simulink model "RoboBoat_SScallv3"  (R2014a)
settings: Solver=FixedStepDiscrete  StartTime=0.0  StopTime=inf  FixedStep=.25  RelTol=1e-3
undefined symbols (not defined in the file): Com1, Com2, Com3, Com4, DiscIntNeverNeededParam, standard
libraries: xpcseriallib x31, visiontextngfix x25, simulink x19, slrtlib x9, speedgoatlib_IO102 x3, speedgoatlib x2
(part 3 of 5)

== system RoboBoat_SScallv3/Main FSM/Obstacle Navigation1/Exit Gate/Gate 1 (Red & White) ==
  Sensors : Inport
  RGB image : Inport  Port=2
  Enable : EnablePort  ShowOutputPort=on
  Bus Selector : BusSelector  OutputSignals=Serial In.Buoy Info.Probability,Serial In.Buoy Info.Color ID,Serial In.Buoy Info.Distance,Serial In.Buoy Info.Angle,Serial In.Compass.Heading,Serial In.GPS.latitude,Serial In.GPS.longitude
  Compare To Constant : simulink/Logic and Bit Operations/Compare To Constant  relop=<=  const=2  OutDataTypeStr=boolean
  Compare To Constant1 : simulink/Logic and Bit Operations/Compare To Constant  relop=>=  const=120  OutDataTypeStr=boolean
  Data Type Conversion2 : DataTypeConversion  OutDataTypeStr=double
  Discrete-Time Integrator : DiscreteIntegrator  SampleTime=.1  ICPrevOutput=DiscIntNeverNeededParam  ICPrevScaledInput=DiscIntNeverNeededParam
  Distance : MATLAB Function  TreatAsAtomicUnit=on
  Insert Text : visiontextngfix/Insert Text  inputType=Obsolete  theText='Exit Gate 1'  getTextLocFrom=Specify via dialog  textLoc=[1 1]  getTextColorFrom=Specify via dialog  textColor=[0 0 0]  getTextIntensityFrom=Specify via dialog  textIntensity=0  getTextOpacityFrom=Specify via dialog  textOpacity=1.0  dummyVar2=0  dummyVar3=0  dummyVar4=0  imagePorts=One multidimensional signal  isInputTransposed=off  fontFace=LucidaSansRegular  dummyVar1=0  blockFontSize=12  antiAliased=on
  Logical Operator : Logic  Operator=OR  AllPortsSameDT=off  OutDataTypeStr=boolean
  MATLAB Function : MATLAB Function  TreatAsAtomicUnit=on
  Output Heirarchy : Subsystem
  Outputs : Outport
  wires:
  Output Heirarchy/1(Outputs) -> Outputs/1
  Sensors/1 -> Output Heirarchy/2(Sensors), Bus Selector/1
  Bus Selector/1 -> MATLAB Function/1(Prob)  "<Probability>"
  Bus Selector/2 -> MATLAB Function/2(ColorID)  "<Color ID>"
  Bus Selector/3 -> MATLAB Function/3(Dist)  "<Distance>"
  Bus Selector/4 -> MATLAB Function/4(Ang)  "<Angle>"
  Bus Selector/5 -> MATLAB Function/5(CurrentHeading)  "<Heading>"
  Enable/1 -> Discrete-Time Integrator/1
  Discrete-Time Integrator/1 -> Compare To Constant1/1, MATLAB Function/8(Timer)
  MATLAB Function/1(RPM) -> Output Heirarchy/3(RPM)
  MATLAB Function/2(DesiredHeading) -> Output Heirarchy/4(Desired Heading)
  Bus Selector/6 -> MATLAB Function/6(GPSLat), Distance/2(GPSLat)  "<latitude>"
  Bus Selector/7 -> MATLAB Function/7(GPSLong), Distance/3(GPSLong)  "<longitude>"
  Distance/1(Distance) -> Compare To Constant/1
  RGB image/1 -> Insert Text/1
  Insert Text/1 -> Output Heirarchy/1(Annotated Image)
  Data Type Conversion2/1 -> Output Heirarchy/5(Task Finished)
  Compare To Constant/1 -> Logical Operator/2
  MATLAB Function/3(gateGPS) -> Distance/1(DesiredGPS)
  Compare To Constant1/1 -> Logical Operator/1
  Logical Operator/1 -> Data Type Conversion2/1

== system RoboBoat_SScallv3/Main FSM/Obstacle Navigation1/Exit Gate/Gate 2 (White & White) ==
  Sensors : Inport
  RGB image : Inport  Port=2
  Enable : EnablePort  ShowOutputPort=on
  Bus Selector : BusSelector  OutputSignals=Serial In.Buoy Info.Probability,Serial In.Buoy Info.Color ID,Serial In.Buoy Info.Distance,Serial In.Buoy Info.Angle,Serial In.Compass.Heading,Serial In.GPS.latitude,Serial In.GPS.longitude
  Compare To Constant : simulink/Logic and Bit Operations/Compare To Constant  relop=<=  const=2  OutDataTypeStr=boolean
  Compare To Constant1 : simulink/Logic and Bit Operations/Compare To Constant  relop=>=  const=120  OutDataTypeStr=boolean
  Data Type Conversion2 : DataTypeConversion  OutDataTypeStr=double
  Discrete-Time Integrator : DiscreteIntegrator  SampleTime=.1  ICPrevOutput=DiscIntNeverNeededParam  ICPrevScaledInput=DiscIntNeverNeededParam
  Distance : MATLAB Function  TreatAsAtomicUnit=on
  Insert Text : visiontextngfix/Insert Text  inputType=Obsolete  theText='Exit Gate 2'  getTextLocFrom=Specify via dialog  textLoc=[1 1]  getTextColorFrom=Specify via dialog  textColor=[0 0 0]  getTextIntensityFrom=Specify via dialog  textIntensity=0  getTextOpacityFrom=Specify via dialog  textOpacity=1.0  dummyVar2=0  dummyVar3=0  dummyVar4=0  imagePorts=One multidimensional signal  isInputTransposed=off  fontFace=LucidaSansRegular  dummyVar1=0  blockFontSize=12  antiAliased=on
  Logical Operator : Logic  Operator=OR  AllPortsSameDT=off  OutDataTypeStr=boolean
  MATLAB Function : MATLAB Function  TreatAsAtomicUnit=on
  Output Heirarchy : Subsystem
  Outputs : Outport
  wires:
  Output Heirarchy/1(Outputs) -> Outputs/1
  Sensors/1 -> Output Heirarchy/2(Sensors), Bus Selector/1
  Bus Selector/1 -> MATLAB Function/1(Prob)  "<Probability>"
  Bus Selector/2 -> MATLAB Function/2(ColorID)  "<Color ID>"
  Bus Selector/3 -> MATLAB Function/3(Dist)  "<Distance>"
  Bus Selector/4 -> MATLAB Function/4(Ang)  "<Angle>"
  Bus Selector/5 -> MATLAB Function/5(CurrentHeading)  "<Heading>"
  Enable/1 -> Discrete-Time Integrator/1
  Discrete-Time Integrator/1 -> Compare To Constant1/1, MATLAB Function/8(Timer)
  MATLAB Function/1(RPM) -> Output Heirarchy/3(RPM)
  MATLAB Function/2(DesiredHeading) -> Output Heirarchy/4(Desired Heading)
  Bus Selector/6 -> MATLAB Function/6(GPSLat), Distance/2(GPSLat)  "<latitude>"
  Bus Selector/7 -> MATLAB Function/7(GPSLong), Distance/3(GPSLong)  "<longitude>"
  Distance/1(Distance) -> Compare To Constant/1
  RGB image/1 -> Insert Text/1
  Data Type Conversion2/1 -> Output Heirarchy/5(Task Finished)
  Compare To Constant/1 -> Logical Operator/2
  MATLAB Function/3(gateGPS) -> Distance/1(DesiredGPS)
  Compare To Constant1/1 -> Logical Operator/1
  Logical Operator/1 -> Data Type Conversion2/1
  Insert Text/1 -> Output Heirarchy/1(Annotated Image)

== system RoboBoat_SScallv3/Main FSM/Obstacle Navigation1/Exit Gate/Gate 3 (White & Green) ==
  Sensors : Inport
  RGB image : Inport  Port=2
  Enable : EnablePort  ShowOutputPort=on
  Bus Selector : BusSelector  OutputSignals=Serial In.Buoy Info.Probability,Serial In.Buoy Info.Color ID,Serial In.Buoy Info.Distance,Serial In.Buoy Info.Angle,Serial In.Compass.Heading,Serial In.GPS.latitude,Serial In.GPS.longitude
  Compare To Constant : simulink/Logic and Bit Operations/Compare To Constant  relop=<=  const=2  OutDataTypeStr=boolean
  Compare To Constant1 : simulink/Logic and Bit Operations/Compare To Constant  relop=>=  const=120  OutDataTypeStr=boolean
  Data Type Conversion2 : DataTypeConversion  OutDataTypeStr=double
  Discrete-Time Integrator : DiscreteIntegrator  SampleTime=.1  ICPrevOutput=DiscIntNeverNeededParam  ICPrevScaledInput=DiscIntNeverNeededParam
  Distance : MATLAB Function  TreatAsAtomicUnit=on
  Insert Text : visiontextngfix/Insert Text  inputType=Obsolete  theText='Exit Gate 3'  getTextLocFrom=Specify via dialog  textLoc=[1 1]  getTextColorFrom=Specify via dialog  textColor=[0 0 0]  getTextIntensityFrom=Specify via dialog  textIntensity=0  getTextOpacityFrom=Specify via dialog  textOpacity=1.0  dummyVar2=0  dummyVar3=0  dummyVar4=0  imagePorts=One multidimensional signal  isInputTransposed=off  fontFace=LucidaSansRegular  dummyVar1=0  blockFontSize=12  antiAliased=on
  Logical Operator : Logic  Operator=OR  AllPortsSameDT=off  OutDataTypeStr=boolean
  MATLAB Function : MATLAB Function  TreatAsAtomicUnit=on
  Output Heirarchy : Subsystem
  Outputs : Outport
  wires:
  Output Heirarchy/1(Outputs) -> Outputs/1
  Sensors/1 -> Output Heirarchy/2(Sensors), Bus Selector/1
  Bus Selector/1 -> MATLAB Function/1(Prob)  "<Probability>"
  Bus Selector/2 -> MATLAB Function/2(ColorID)  "<Color ID>"
  Bus Selector/3 -> MATLAB Function/3(Dist)  "<Distance>"
  Bus Selector/4 -> MATLAB Function/4(Ang)  "<Angle>"
  Bus Selector/5 -> MATLAB Function/5(CurrentHeading)  "<Heading>"
  Enable/1 -> Discrete-Time Integrator/1
  Discrete-Time Integrator/1 -> Compare To Constant1/1, MATLAB Function/8(Timer)
  MATLAB Function/1(RPM) -> Output Heirarchy/3(RPM)
  MATLAB Function/2(DesiredHeading) -> Output Heirarchy/4(Desired Heading)
  Bus Selector/6 -> MATLAB Function/6(GPSLat), Distance/2(GPSLat)  "<latitude>"
  Bus Selector/7 -> MATLAB Function/7(GPSLong), Distance/3(GPSLong)  "<longitude>"
  Distance/1(Distance) -> Compare To Constant/1
  RGB image/1 -> Insert Text/1
  Data Type Conversion2/1 -> Output Heirarchy/5(Task Finished)
  Compare To Constant/1 -> Logical Operator/2
  MATLAB Function/3(gateGPS) -> Distance/1(DesiredGPS)
  Compare To Constant1/1 -> Logical Operator/1
  Logical Operator/1 -> Data Type Conversion2/1
  Insert Text/1 -> Output Heirarchy/1(Annotated Image)

== system RoboBoat_SScallv3/Main FSM/Obstacle Navigation1/GPS: Center/Approach ==
  Sensors : Inport
  RGB image : Inport  Port=2
  Enable : EnablePort
  Annotate Task : visiontextngfix/Insert Text  inputType=Obsolete  theText='GPS - Center: Approach - Distance: %f'  getTextLocFrom=Specify via dialog  textLoc=[10 70]  getTextColorFrom=Specify via dialog  textColor=[255 0 0]  getTextIntensityFrom=Specify via dialog  textIntensity=0  getTextOpacityFrom=Specify via dialog  textOpacity=1.0  dummyVar2=0  dummyVar3=0  dummyVar4=0  imagePorts=One multidimensional signal  isInputTransposed=off  fontFace=LucidaSansRegular  dummyVar1=0  blockFontSize=12  antiAliased=on
  Annotate Task2 : visiontextngfix/Insert Text  inputType=Obsolete  theText='Obst Nav Start'  getTextLocFrom=Specify via dialog  textLoc=[1 1]  getTextColorFrom=Specify via dialog  textColor=[0 0 0]  getTextIntensityFrom=Specify via dialog  textIntensity=0  getTextOpacityFrom=Specify via dialog  textOpacity=1.0  dummyVar2=0  dummyVar3=0  dummyVar4=0  imagePorts=One multidimensional signal  isInputTransposed=off  fontFace=LucidaSansRegular  dummyVar1=0  blockFontSize=12  antiAliased=on
  Bus Selector : BusSelector  OutputSignals=Serial In.GPS.latitude,Serial In.GPS.longitude
  Compare To Constant : simulink/Logic and Bit Operations/Compare To Constant  relop=<=  const=5  OutDataTypeStr=boolean
  Data Store Read : DataStoreRead  DataStoreName=obstNavStartGPS  SampleTime=0.1
  Data Type Conversion : DataTypeConversion  OutDataTypeStr=double
  Desired Heading and Distance : MATLAB Function  TreatAsAtomicUnit=on
  MATLAB Function : MATLAB Function  Commented=on  TreatAsAtomicUnit=on
  Output Heirarchy : Subsystem
  "Scope " : slrtlib/Displays and Logging/Scope   Commented=on  scopeno=1  scopetype=File  autostart=on  viewmode=Graphical redraw  formatstr='%15.6f'  grid=on  ylimits=[0,0]  nosamples=1200  noprepostsamples=0  interleave=1  triggermode=FreeRun  triggersignal=1  trigsignalfromport=off  triggerlevel=1  triggerslope=Either  triggerscope=1  triggersample=0  filename=ApprLog.dat  mode=Lazy  writesize=512  autorestart=off  dynamicfilemode=off  maxwritefilesize=512*1024^2
  Outputs : Outport
  wires:
  Sensors/1 -> Output Heirarchy/4(Sensors), Bus Selector/1  "Sensors"
  Data Store Read/1 -> Desired Heading and Distance/1(DesiredGPS)
  Bus Selector/1 -> Desired Heading and Distance/2(GPSLat)  "<latitude>"
  Bus Selector/2 -> Desired Heading and Distance/3(GPSLong)  "<longitude>"
  Desired Heading and Distance/2(DesiredHeading) -> Output Heirarchy/2(Desired Heading)
  Annotate Task/1 -> Output Heirarchy/3(Annotated Image)
  RGB image/1 -> Annotate Task2/1
  Output Heirarchy/1(Outputs) -> Outputs/1
  Annotate Task2/1 -> Annotate Task/1
  MATLAB Function/1(out) -> "Scope "/1
  Desired Heading and Distance/1(Distance) -> Compare To Constant/1, Annotate Task/2
  Data Type Conversion/1 -> Output Heirarchy/1(Finished)  "Task Finished"
  Compare To Constant/1 -> Data Type Conversion/1

== system RoboBoat_SScallv3/Main FSM/Obstacle Navigation1/GPS: Center/Orient ==
  Sensors : Inport
  RGB image : Inport  Port=2
  Enable : EnablePort
  Annotate Task : visiontextngfix/Insert Text  inputType=Obsolete  theText='GPS - Center: Orient %f'  getTextLocFrom=Specify via dialog  textLoc=[10 70]  getTextColorFrom=Specify via dialog  textColor=[255 0 0]  getTextIntensityFrom=Specify via dialog  textIntensity=0  getTextOpacityFrom=Specify via dialog  textOpacity=1.0  dummyVar2=0  dummyVar3=0  dummyVar4=0  imagePorts=One multidimensional signal  isInputTransposed=off  fontFace=LucidaSansRegular  dummyVar1=0  blockFontSize=12  antiAliased=on
  Annotate Task1 : visiontextngfix/Insert Text  inputType=Obsolete  theText='Current Heading %f'  getTextLocFrom=Specify via dialog  textLoc=[10 40]  getTextColorFrom=Specify via dialog  textColor=[255 0 0]  getTextIntensityFrom=Specify via dialog  textIntensity=0  getTextOpacityFrom=Specify via dialog  textOpacity=1.0  dummyVar2=0  dummyVar3=0  dummyVar4=0  imagePorts=One multidimensional signal  isInputTransposed=off  fontFace=LucidaSansRegular  dummyVar1=0  blockFontSize=12  antiAliased=on
  Annotate Task2 : visiontextngfix/Insert Text  inputType=Obsolete  theText='Obst Nav Start'  getTextLocFrom=Specify via dialog  textLoc=[1 1]  getTextColorFrom=Specify via dialog  textColor=[0 0 0]  getTextIntensityFrom=Specify via dialog  textIntensity=0  getTextOpacityFrom=Specify via dialog  textOpacity=1.0  dummyVar2=0  dummyVar3=0  dummyVar4=0  imagePorts=One multidimensional signal  isInputTransposed=off  fontFace=LucidaSansRegular  dummyVar1=0  blockFontSize=12  antiAliased=on
  Bus Selector : BusSelector  OutputSignals=Serial In.GPS.latitude,Serial In.GPS.longitude,Serial In.Compass.Heading
  Data Store Read : DataStoreRead  DataStoreName=obstNavStartGPS  SampleTime=0.1
  Desired Heading : MATLAB Function  TreatAsAtomicUnit=on
  Output Heirarchy1 : Subsystem
  Within Range : MATLAB Function  TreatAsAtomicUnit=on
  Outputs : Outport
  Finished : Outport  Port=2
  wires:
  Sensors/1 -> Output Heirarchy1/3(Sensors), Bus Selector/1  "Sensors"
  Data Store Read/1 -> Desired Heading/1(DesiredGPS)
  Bus Selector/1 -> Desired Heading/2(GPSLat)  "<latitude>"
  Bus Selector/2 -> Desired Heading/3(GPSLong)  "<longitude>"
  Desired Heading/1(DesiredHeading) -> Output Heirarchy1/2(Desired Heading), Annotate Task/2, Within Range/1(DesiredHeading)
  Bus Selector/3 -> Annotate Task1/2, Within Range/2(Compass)  "<Heading>"
  Within Range/1(Finished) -> Finished/1
  RGB image/1 -> Annotate Task2/1
  Output Heirarchy1/1(Outputs) -> Outputs/1
  Annotate Task/1 -> Annotate Task1/1
  Annotate Task1/1 -> Output Heirarchy1/1(Annotated Image)
  Annotate Task2/1 -> Annotate Task/1

== system RoboBoat_SScallv3/Main FSM/Obstacle Navigation1/GPS: Center/Output Reassign ==
  Outputs in : Inport
  Bus Assignment : BusAssignment  AssignedSignals=Task Finished
  Bus Selector : BusSelector  OutputSignals=Task Finished
  Constant : Constant  Value=0
  Outputs : Outport
  Finished : Outport  Port=2
  wires:
  Outputs in/1 -> Bus Assignment/1, Bus Selector/1
  Bus Selector/1 -> Finished/1  "<Task Finished>"
  Bus Assignment/1 -> Outputs/1
  Constant/1 -> Bus Assignment/2

== matlab function RoboBoat_SScallv3/Main FSM/Obstacle Navigation1/Exit Gate/Gate 3 (White & Green)/Distance ==
  data: Distance output; DesiredGPS input; GPSLat input; GPSLong input
function Distance  = DistCalc(DesiredGPS, GPSLat, GPSLong)

%Written by Anderson Lebbad on July 22, 2013
%Last Edited:

%Orients the boat towards a target GPS point before approaching it.
%This is done to keep the approach angle minimal, so the approach
%algorithm does not circle the target and never reach it.

%Parse input GPS and convert angles to radians
CurLat = (floor(GPSLat/100)+mod(GPSLat,100)/60)*pi/180;
CurLong = (floor(GPSLong/100)+mod(GPSLong,100)/60)*pi/180;
DesLat = (floor(DesiredGPS(1)/100)+mod(DesiredGPS(1),100)/60)*pi/180;
DesLong = (floor(DesiredGPS(2)/100)+mod(DesiredGPS(2),100)/60)*pi/180;
%Difference between lats and longs
DiffLat = DesLat - CurLat;
MidLat = cos((CurLat + DesLat)/2);
DiffLong = DesLong - CurLong;
%Radius of the earth in meters
R = 6378137;

%Calculate distance using the great-circle distance formula
%Formula documented here:
%   http://www.movable-type.co.uk/scripts/latlong.html
% a = sin(DiffLat/2)^2+sin(DiffLong/2)^2*cos(CurLat)*cos(DesLat);
% c = 2*atan2(sqrt(a), sqrt(1-a));
% Distance = R*c;

%Calculating distance using Pythagora's
a = DiffLong*MidLat;
b = DiffLat;
Distance = R*sqrt(a^2+b^2);

== matlab function RoboBoat_SScallv3/Main FSM/Obstacle Navigation1/Exit Gate/MATLAB Function ==
  data: gateID input; outputSelector output; gate1En output; gate2En output; gate3En output
function [outputSelector,gate1En,gate2En,gate3En] = gateSelector(gateID)
% Determines which colors to filter for based on the gateID as received
% from the judges

gate1En = 0;
gate2En = 0;
gate3En = 0;

if gateID == 1
    gate1En = 1;
    outputSelector = 1;
elseif gateID == 2
    gate2En = 1;
    outputSelector = 2;
else
    gate3En = 1;
    outputSelector = 3;
end

== matlab function RoboBoat_SScallv3/Sinks/actuators/analog output/Subsystem/Heading Controller/MATLAB Function ==
  data: HeadingDesired input; steering output; CompassHeading input
function steering = CalcSteering(HeadingDesired, CompassHeading)

%Written by Anderson Lebbad on May 29, 2015
%Last Edited: Anderson Lebbad on June 7, 2015
%   Simplified using mod division

%Calculates the difference between the desired and current heading to be
%used for steering

steering = HeadingDesired - CompassHeading;
%atan2 in radians, input and output in degrees
steering = atan2(sin(steering*pi/180),cos(steering*pi/180))*180/pi;

== matlab function RoboBoat_SScallv3/Main FSM/Start Speed/Gate Find and Through/Find/MATLAB Function1 ==
  data: Dist input; Angles input; X input; Y input; Heading input; found output; Goal output; DesiredHeading output
function [found, Goal, DesiredHeading] = SpeedGate(Dist,Angles,X,Y,Heading)
%Written by Anderson Lebbad on May 29, 2015
%Last Edited by:

%This function sends theboat forward until a landmark is found, then it
%navigates towards the right of it.

persistent goalX goalY Found initialHeading change
if isempty(goalX)
    goalX = X;
    goalY = Y;
    Found = 0;
    initialHeading = Heading;
    change = 10;
end

DesiredHeading = Heading;
DistM = Dist./100;
dodgeWidth = 3;

if Found == 0
    if DistM(2) ~= 0
        %If two objects are found, set goal between the two
        w = (DistM(1)*sin(Angles(1)) + DistM(2)*sin(Angles(2)*pi/180)) / 2;
        h = (DistM(1)*cos(Angles(1)) + DistM(2)*sin(Angles(2)*pi/180)) / 2;
        goalX = X + h*cos(Heading) - w*sin(Heading);
        goalY = Y + h*sin(Heading) + w*cos(Heading);
        Found = 1;
    elseif DistM(1) ~= 0
        %If one object is found, set goal dodgewidth to the right of it
        w = DistM(1)*sin(Angles(1)) + dodgeWidth;
        h = DistM(1)*cos(Angles(1));
        goalX = X + h*cos(Heading) - w*sin(Heading);
        goalY = Y + h*sin(Heading) + w*cos(Heading);
        Found = 1;
    else
        %If no objects are found, search. Scan 30 degrees to left and right
        %of initial heading.
        DesiredHeading = Heading + change;
        if abs(DesiredHeading - initialHeading) > 30
            change = -change;
            DesiredHeading = Heading + change;
        end
    end
end

Goal = [goalX, goalY];
found = Found;

end

== matlab function RoboBoat_SScallv3/Main FSM/Obstacle Navigation1/Enter Gate/Gate 1 (Red & White)/MATLAB Function ==
  data: Prob input; RPM output; ColorID input; Dist input; Ang input; CurrentHeading input; GPSLat input; GPSLong input; Timer input; DesiredHeading output; gateGPS output
function [RPM,DesiredHeading,gateGPS] = navigation(Prob,ColorID,Dist,Ang,CurrentHeading,GPSLat,GPSLong,Timer)

% Function performs one buoy navigation through the start speed gates. If
% no buoys are found by the LIDAR/Vision assembly then an incremented
% turning algorithm is executed to turn by 10 degrees per increment up to 
% 90 degrees either way of the inital heading

% Written by Edward Zhu

persistent LockHeading TimeLastFound Counter Turn TurnInc gateLat gateLong

if isempty(LockHeading) && isempty(TimeLastFound) && isempty(Counter) && isempty(Turn) && isempty(TurnInc)
    LockHeading = CurrentHeading;
    TimeLastFound = 0;
    Counter = 0;
    TurnInc = 30;
    Turn = TurnInc;
    gateLat = 0;
    gateLong = 0;
end

Distance = Dist/100;

BoatWidth = 0.75;
Buffer = atan(2*BoatWidth/Distance);

RedOffset = Ang + Buffer;
WhiteOffset = Ang - Buffer;

R = 6378137;

CurLat = (floor(GPSLat/100)+mod(GPSLat,100)/60)*pi/180;
CurLong = (ceil(GPSLong/100)-mod(-GPSLong,100)/60)*pi/180;

gateHeading = (mod(CurrentHeading + Ang, 360))*pi/180;

if ColorID == 1 && Prob > 0.9
    if Ang < 0
        DesiredHeading = mod(CurrentHeading - RedOffset, 360);
    else
        DesiredHeading = mod(CurrentHeading + RedOffset, 360);
    end
    RPM = 4000;
    GateFound = 1;
    TimeLastFound = Timer;
    gateLat =  asin(sin(CurLat)*cos(Distance/R) + cos(CurLat)*sin(Distance/R)*cos(gateHeading))*180/pi;
    gateLong = (CurLong + atan2(sin(gateHeading)*sin(Distance/R)*cos(CurLat),cos(Distance/R)-sin(CurLat)*sin(gateLat)))*180/pi;
elseif ColorID == 2 && Prob > 0.9
    DesiredHeading = mod(LockHeading - Turn, 360);
    RPM = 0;
    GateFound = 1;
    TimeLastFound = Timer;
%     DesiredHeading = mod(CurrentHeading - WhiteOffset, 360);
%     RPM = 4000;
%     GateFound = 1;
%     TimeLastFound = Timer;
%     gateLat =  asin(sin(CurLat)*cos(Distance/R) + cos(CurLat)*sin(Distance/R)*cos(gateHeading))*180/pi;
%     gateLong = (CurLong + atan2(sin(gateHeading)*sin(Distance/R)*cos(CurLat),cos(Distance/R)-sin(CurLat)*sin(gateLat)))*180/pi;
else
    DesiredHeading = CurrentHeading;
    RPM = 0;
    GateFound = 0;
end

gateGPS = [gateLat gateLong];
TimeNoBuoys = Timer - TimeLastFound;

if GateFound == 0 && TimeNoBuoys > 15
    RPM = 0;
    DesiredHeading = mod(LockHeading - Turn, 360);
    HeadingDiff = DesiredHeading - CurrentHeading;
    gateGPS = [gateLat gateLong];
    
    if HeadingDiff > 180
        HeadingDiff = HeadingDiff - 360;
    elseif HeadingDiff < -180
        HeadingDiff = HeadingDiff + 360;
    end
    
    if HeadingDiff < 3
        Counter = Counter + 1;
    else
        Counter = 0;
    end
    
    if Counter >= 15
        Turn = Turn + TurnInc;
        Counter = 0;
        if abs(Turn) > 90
            TurnInc = -TurnInc;
        end
    end
end

== matlab function RoboBoat_SScallv3/Main FSM/Start Speed/Gate Find and Through1/GPS Enabler ==
  data: Finished input; GPSMode output; OrientEn output; ApproachEn output
function [GPSMode, OrientEn, ApproachEn] = GPSEnable(Finished)

%Written by Anderson Lebbad on July 22, 2013
%Last Edited: July 27, 2013
%   Removed Termination Block

%This function enables GPS tasks. First the boat orients towards the
%target, then it approaches it.


%Parse Finished signal
OrientFinished = Finished(1);


%Initialize Enablers
OrientEn = 0;
ApproachEn = 0;


%Switches the enable signal based on which task is flagged as done.
if OrientFinished == 0
    OrientEn = 1;
    GPSMode = 1;
else
    ApproachEn = 1;
    GPSMode = 2;
end

== matlab function RoboBoat_SScallv3/Main FSM/Obstacle Navigation1/Obstacle Navigation/GPS: Bee Line/Orient/Desired Heading ==
  data: DesiredGPS input; DesiredHeading output; GPSLat input; GPSLong input
function DesiredHeading = Orient(DesiredGPS, GPSLat, GPSLong)

%Written by Anderson Lebbad on July 22, 2013
%Last Edited: Edward Zhu on July 5, 2014

% Edit:
% Changed calculation to use positive lat and negative long

%Orients the boat towards a target GPS point before approaching it.
%This is done to keep the approach angle minimal, so the approach
%algorithm does not circle the target and never reach it.

%Parse input GPS and convert angles to radians
CurLat = (floor(GPSLat/100)+mod(GPSLat,100)/60)*pi/180;
CurLong = (ceil(GPSLong/100)-mod(-GPSLong,100)/60)*pi/180;
DesLat = (floor(DesiredGPS(1)/100)+mod(DesiredGPS(1),100)/60)*pi/180;
DesLong = (ceil(DesiredGPS(2)/100)-mod(-DesiredGPS(2),100)/60)*pi/180;

%Difference between longs
DiffLong = DesLong - CurLong;

%Calculate initial bearing - formula documented here: 
%   http://www.movable-type.co.uk/scripts/latlong.html
y = sin(DiffLong)*cos(DesLat);
x = cos(CurLat)*sin(DesLat)-sin(CurLat)*cos(DesLat)*cos(DiffLong);
DesiredHeading = mod(atan2(y, x)*180/pi + 360, 360);

== matlab function RoboBoat_SScallv3/Main FSM/Obstacle Navigation1/GPS: Center/Approach/MATLAB Function ==
  data: GPSLat input; out output; GPSLong input; IMULat input; IMULong input
function out = dataFormat(GPSLat, GPSLong, IMULat, IMULong)
%#codegen
out = [GPSLat GPSLong IMULat IMULong];

== matlab function RoboBoat_SScallv3/Main FSM/Obstacle Navigation1/GPS: Center/Orient/Desired Heading ==
  data: DesiredGPS input; DesiredHeading output; GPSLat input; GPSLong input
function DesiredHeading = Orient(DesiredGPS, GPSLat, GPSLong)

%Written by Anderson Lebbad on July 22, 2013
%Last Edited: Edward Zhu on July 5, 2014

% Edit:
% Changed calculation to use positive lat and negative long

%Orients the boat towards a target GPS point before approaching it.
%This is done to keep the approach angle minimal, so the approach
%algorithm does not circle the target and never reach it.

%Parse input GPS and convert angles to radians
CurLat = (floor(GPSLat/100)+mod(GPSLat,100)/60)*pi/180;
CurLong = (ceil(GPSLong/100)-mod(-GPSLong,100)/60)*pi/180;
DesLat = (floor(DesiredGPS(1)/100)+mod(DesiredGPS(1),100)/60)*pi/180;
DesLong = (ceil(DesiredGPS(2)/100)-mod(-DesiredGPS(2),100)/60)*pi/180;

%Difference between longs
DiffLong = DesLong - CurLong;

%Calculate initial bearing - formula documented here: 
%   http://www.movable-type.co.uk/scripts/latlong.html
y = sin(DiffLong)*cos(DesLat);
x = cos(CurLat)*sin(DesLat)-sin(CurLat)*cos(DesLat)*cos(DiffLong);
DesiredHeading = mod(atan2(y, x)*180/pi + 360, 360);

== matlab function RoboBoat_SScallv3/Main FSM/Obstacle Navigation1/MATLAB Function1 ==
  data: taskMode input; taskSelector output; startGPSFin input; commFin input; enterGateFin input; obstNavFin input; startGPSEn output; commEn output; enterGateEn output; obstNavEn output; exitGateEn output
function [taskSelector,startGPSEn,commEn,enterGateEn,obstNavEn,exitGateEn]...
    = taskEnabler(taskMode,startGPSFin,commFin,enterGateFin,obstNavFin)

startGPSEn = 0;
commEn = 0;
enterGateEn = 0;
obstNavEn = 0;
exitGateEn = 0;

taskOption = char(taskMode);

if ~isempty(strfind(taskOption,'Comm'))
    startGPSFin = 1;
elseif ~isempty(strfind(taskOption,'Enter'))
    startGPSFin = 1;
    commFin = 1;
elseif ~isempty(strfind(taskOption,'Nav'))
    startGPSFin = 1;
    commFin = 1;
    enterGateFin = 1;
elseif ~isempty(strfind(taskOption,'Exit'))
    startGPSFin = 1;
    commFin = 1;
    enterGateFin = 1;
    obstNavFin = 1;
end

if startGPSFin == 0
    startGPSEn = 1;
    taskSelector = 1;
elseif commFin == 0
    commEn = 1;
    taskSelector = 2;
elseif enterGateFin == 0
    enterGateEn = 1;
    taskSelector = 3;
elseif obstNavFin == 0
    obstNavEn = 1;
    taskSelector = 4;
else
    exitGateEn = 1;
    taskSelector = 5;
end

== matlab function RoboBoat_SScallv3/Main FSM/Obstacle Navigation1/Obstacle Navigation/GPS: Bee Line/Approach/Obstacle Distance ==
  data: ColorID input; ObstDist output; DodgeStart output; Dist input
function [ObstDist, DodgeStart] = obstDist(ColorID,Dist)

%Written by Edward Zhu
%Last Edited by:

ObstDist = Dist / 100;

% if ColorID == 5 || ColorID == 6
    if ObstDist <= 3
        DodgeStart = 1;
    else
        DodgeStart = 0;
    end
% else
%     DodgeStart = 0;
% end

== matlab function RoboBoat_SScallv3/Main FSM/Obstacle Navigation1/Obstacle Navigation/GPS: Bee Line/GPS Enabler ==
  data: Finished input; GPSMode output; OrientEnable output; ApproachEnable output
function [GPSMode, OrientEnable, ApproachEnable] =...
    GPSEnable(Finished)

%Written by Anderson Lebbad on July 22, 2013
%Last Edited: July 27, 2013
%   Removed Termination Block

%This function enables GPS tasks. First the boat orients towards the
%target, then it approaches it.


%Parse Finished signal
OrientFinished = Finished(1);


%Initialize Enablers
OrientEnable = 0;
ApproachEnable = 0;


%Switches the enable signal based on which task is flagged as done.
if OrientFinished == 0
    OrientEnable = 1;
    GPSMode = 1;
else
    ApproachEnable = 1;
    GPSMode = 2;
end

== matlab function RoboBoat_SScallv3/Sensors/1020 Comms/MATLAB Function1 ==
  data: Valid input; Time input; asciiSEA output; Lat input; Long input; Color input; Depth input
% This function creates the underwater search message to be sent from 
% Speedgoat in ascii code
% Written by: Edward Zhu
% Date: 9/17/14

function asciiSEA = asciiSEAEncoder(Valid, Time, Lat, Long, Color, Depth)

% Initialize output message vector as the serial output block expects 128
% character message
asciiSEA = uint8(zeros(1,128));

% Convert static strings to ascii code
asciiMsgID = uint8('$RXSEA,');
asciiComma = uint8(',');
asciiDeciPt = uint8('.');
if Valid == 1
    if Lat >= 0
        asciiNS = uint8('N,');
    else
        Lat = -Lat;
        asciiNS = uint8('S,');
    end
    if Long >= 0
        asciiEW = uint8('E,');
    else
        Long = -Long;
        asciiEW = uint8('W,');
    end
else
    asciiNS = [32 asciiComma];
    asciiEW = [32 asciiComma];
end
asciiTeamID = uint8('FAUVU,');
asciiMsgEnd = uint8('*');
asciiMsgCRLF = [13 10];

% Convert UTC Time input (hhmmss) into ascii code
asciiTime = uint8(zeros(1,7));
asciiTime(7) = asciiComma;

for timeChar = 1:6
    asciiTime(timeChar) = floor(mod(Time,10^(7-timeChar))/...
        10^(6-timeChar)) + 48;
end

% Convert buoy color to ascii code (1 = R, 2 = G, 3 = B, 4 = W, 5 = K)
asciiColor = [uint8(32) asciiComma]; % Initialize as whitespace in case no buoy is found
if Valid == 1
    if Color == 1
        asciiColor(1) = uint8('R');
    elseif Color == 2
        asciiColor(1) = uint8('G');
    elseif Color == 3
        asciiColor(1) = uint8('B');
    elseif Color == 4
        asciiColor(1) = uint8('W');
    elseif Color == 5
        asciiColor(1) = uint8('K');
    end
end
% Convert latitude (dd.mmmmmm) into ascii code
asciiLat = uint8(zeros(1,10)+32); % Initialize as whitespace in case no buoy is found
asciiLat(10) = asciiComma;

% Only output values if valid bit is high
if Valid == 1
    asciiLat(3) = asciiDeciPt;
    latInt = floor(Lat);
    for latIntChar = 1:2
        asciiLat(latIntChar) = floor(mod(latInt,10^(3-latIntChar))/...
            10^(2-latIntChar)) + 48;
    end
    
    latDeci = mod(Lat,latInt) * 10^6;
    for latDeciChar = 1:6
        asciiLat(latDeciChar+3) = floor(mod(latDeci,10^(7-latDeciChar))/...
            10^(6-latDeciChar)) + 48;
    end
end

% Convert longitude (ddd.mmmmmm) into ascii code
asciiLong = uint8(zeros(1,11)+32); % Initialize as whitespace in case no buoy is found
asciiLong(11) = asciiComma;

% Only output values if valid bit is high
if Valid == 1
    asciiLong(4) = asciiDeciPt;
    longInt = floor(Long);
    for longIntChar = 1:3
        asciiLong(longIntChar) = floor(mod(longInt,10^(4-longIntChar))/...
            10^(3-longIntChar)) + 48;
    end
    
    longDeci = mod(Long,longInt) * 10^6;
    for longDeciChar = 1:6
        asciiLong(longDeciChar+4) = floor(mod(longDeci,10^(7-longDeciChar))/...
            10^(6-longDeciChar)) + 48;
    end
end

% Convert depth (m) (##.##) into ascii
asciiDepth = uint8(zeros(1,6)+32); % Initialize as whitespace in case no buoy is found
asciiDepth(6) = asciiMsgEnd;

% Only output values if valid bit is high
if Valid == 1
    asciiDepth(3) = asciiDeciPt;
    depthInt = floor(Depth);
    for depthIntChar = 1:2
        asciiDepth(depthIntChar) = floor(mod(depthInt,10^(3-depthIntChar))/...
            10^(2-depthIntChar)) + 48;
    end
    
    depthDeci = mod(Depth,depthInt) * 10^2;
    for depthDeciChar = 1:2
        asciiDepth(depthDeciChar+3) = floor(mod(depthDeci,10^(3-depthDeciChar))/...
            10^(2-depthDeciChar)) + 48;
    end
end

% Concat individual ascii arrays into one array
asciiPreChkSum = cat(2,asciiMsgID,asciiTime,asciiTeamID,asciiColor,...
    asciiLat,asciiNS,asciiLong,asciiEW,asciiDepth);

% Calculate the checksum of the message from the '$' to the '*' and convert
% to hex
chkSum = uint8(0);

for chksumChar = 1:(length(asciiPreChkSum)-2)
    chkSum = bitxor(chkSum,asciiPreChkSum(chksumChar+1));
end

% Convert the checksum to ascii
chkSum = dec2hex(chkSum);
asciiChkSum = uint8(zeros(1,length(chkSum))+32);
for i = 1:length(chkSum)
    asciiChkSum(i) = uint8(chkSum(i));
end

% Concat the checksum and the '/r/n' to the end of the message
asciiPostChkSum = cat(2,asciiPreChkSum,asciiChkSum,asciiMsgCRLF);

% Output the final message
asciiSEA(1:length(asciiPostChkSum)) = asciiPostChkSum;

== system RoboBoat_SScallv3/Main FSM/Obstacle Navigation1/Obstacle Navigation/Dodge ==
  Sensors : Inport
  RGB image : Inport  Port=2
  Enable : EnablePort  ShowOutputPort=on
  Bus Selector1 : BusSelector  OutputSignals=Serial In.Compass.Heading,Serial In.Buoy Info.Distance,Serial In.Buoy Info.Angle
  Constant : Constant  Value=0
  Constant1 : Constant  Value=2
  Data Store Write : DataStoreWrite  DataStoreName=dodgeStart
  Discrete-Time Integrator : DiscreteIntegrator  SampleTime=0.1  ICPrevOutput=DiscIntNeverNeededParam  ICPrevScaledInput=DiscIntNeverNeededParam
  Insert Text : visiontextngfix/Insert Text  inputType=Obsolete  theText='Dodge'  getTextLocFrom=Specify via dialog  textLoc=[1 1]  getTextColorFrom=Specify via dialog  textColor=[0 0 0]  getTextIntensityFrom=Specify via dialog  textIntensity=0  getTextOpacityFrom=Specify via dialog  textOpacity=1.0  dummyVar2=0  dummyVar3=0  dummyVar4=0  imagePorts=One multidimensional signal  isInputTransposed=off  fontFace=LucidaSansRegular  dummyVar1=0  blockFontSize=12  antiAliased=on
  Insert Text1 : visiontextngfix/Insert Text  inputType=Obsolete  theText='Obstacle Distance: %f'  getTextLocFrom=Specify via dialog  textLoc=[10 70]  getTextColorFrom=Specify via dialog  textColor=[255 0 0]  getTextIntensityFrom=Specify via dialog  textIntensity=0  getTextOpacityFrom=Specify via dialog  textOpacity=1.0  dummyVar2=0  dummyVar3=0  dummyVar4=0  imagePorts=One multidimensional signal  isInputTransposed=off  fontFace=LucidaSansRegular  dummyVar1=0  blockFontSize=12  antiAliased=on
  Nav Logic : MATLAB Function  TreatAsAtomicUnit=on
  Output Heirarchy : Subsystem
  Unit Delay1 : UnitDelay  InitialCondition=1  SampleTime=-1
  Outputs : Outport
  Dodge Incomplete : Outport  Port=2
  wires:
  RGB image/1 -> Insert Text/1
  Sensors/1 -> Output Heirarchy/2(Sensors), Bus Selector1/1
  Bus Selector1/1 -> Nav Logic/1(CurrentHeading)  "<Heading>"
  Enable/1 -> Discrete-Time Integrator/1
  Discrete-Time Integrator/1 -> Nav Logic/4(Timer)
  Constant1/1 -> Nav Logic/5(Timeout)
  Nav Logic/4(DodgeIncomplete) -> Dodge Incomplete/1
  Insert Text/1 -> Insert Text1/1
  Nav Logic/1(ObstDist) -> Insert Text1/2
  Nav Logic/2(RPM) -> Output Heirarchy/3(RPM)
  Nav Logic/3(DesiredHeading) -> Output Heirarchy/4(Desired Heading)
  Output Heirarchy/1(Outputs) -> Outputs/1
  Constant/1 -> Unit Delay1/1
  Unit Delay1/1 -> Data Store Write/1
  Insert Text1/1 -> Output Heirarchy/1(Annotated Image)
  Bus Selector1/2 -> Nav Logic/2(Dist)  "<Distance>"
  Bus Selector1/3 -> Nav Logic/3(Ang)  "<Angle>"

== system RoboBoat_SScallv3/Main FSM/Obstacle Navigation1/Obstacle Navigation/GPS: Bee Line ==
  Sensors : Inport
  RGB image : Inport  Port=2
  Enable : EnablePort
  Approach : Subsystem  TreatAsAtomicUnit=on
  Data Store Write : DataStoreWrite  DataStoreName=dodgeStart
  GPS Enabler : MATLAB Function  TreatAsAtomicUnit=on
  GPS Selector : MultiPortSwitch  Inputs=2
  Orient : Subsystem  TreatAsAtomicUnit=on
  Unit Delay : UnitDelay  SampleTime=-1
  Unit Delay1 : UnitDelay  SampleTime=-1
  Outputs : Outport
  wires:
  Sensors/1 -> Orient/1(Sensors), Approach/1(Sensors)
  GPS Enabler/2(OrientEnable) -> Orient/Enable
  GPS Enabler/3(ApproachEnable) -> Approach/Enable
  Orient/2(Finished) -> Unit Delay/1
  Orient/1(Outputs) -> GPS Selector/2
  Approach/1(Outputs) -> GPS Selector/3
  GPS Enabler/1(GPSMode) -> GPS Selector/1
  Unit Delay/1 -> GPS Enabler/1(Finished)
  RGB image/1 -> Orient/2(RGB image), Approach/2(RGB image)
  Approach/2(Dodge Start) -> Unit Delay1/1
  Unit Delay1/1 -> Data Store Write/1
  GPS Selector/1 -> Outputs/1

== system RoboBoat_SScallv3/Main FSM/Obstacle Navigation1/Obstacle Navigation/Output Reassign ==
  Outputs in : Inport
  Bus Assignment : BusAssignment  AssignedSignals=Task Finished
  Bus Selector : BusSelector  OutputSignals=Task Finished
  Constant : Constant  Value=0
  Outputs : Outport
  Finished : Outport  Port=2
  wires:
  Outputs in/1 -> Bus Assignment/1, Bus Selector/1
  Bus Selector/1 -> Finished/1  "<Task Finished>"
  Bus Assignment/1 -> Outputs/1
  Constant/1 -> Bus Assignment/2

== system RoboBoat_SScallv3/Main FSM/Start Speed/Gate Find and Through/Find ==
  Sensors : Inport
  Enable : EnablePort
  Bus Selector : BusSelector  OutputSignals=Lidar Data Input.Landmarks.Distances,Lidar Data Input.Landmarks.Angles,GPS.X,GPS.Y,Compass.Heading
  MATLAB Function1 : MATLAB Function  TreatAsAtomicUnit=on
  Output Heirarchy : Subsystem
  RPM : Constant  Value=0  SampleTime=-1
  Write : DataStoreWrite  DataStoreName=GateNED
  Outputs : Outport
  Finished : Outport  Port=2
  wires:
  Output Heirarchy/1(Outputs) -> Outputs/1
  RPM/1 -> Output Heirarchy/2(RPM)
  MATLAB Function1/2(Goal) -> Write/1
  MATLAB Function1/1(found) -> Finished/1
  MATLAB Function1/3(DesiredHeading) -> Output Heirarchy/3(Desired Heading)
  Sensors/1 -> Output Heirarchy/1(Sensors), Bus Selector/1  "Sensors"
  Bus Selector/1 -> MATLAB Function1/1(Dist)  "<Distances>"
  Bus Selector/3 -> MATLAB Function1/3(X)  "<X>"
  Bus Selector/2 -> MATLAB Function1/2(Angles)  "<Angles>"
  Bus Selector/4 -> MATLAB Function1/4(Y)  "<Y>"
  Bus Selector/5 -> MATLAB Function1/5(Heading)  "<Heading>"

== system RoboBoat_SScallv3/Main FSM/Start Speed/Gate Find and Through/Through ==
  Sensors : Inport
  Enable : EnablePort
  Bus Selector2 : BusSelector  OutputSignals=GPS.X,GPS.Y,Compass.Heading
  Data Store Read3 : DataStoreRead  DataStoreName=GateNED
  Demux : Demux  Outputs=2
  Model : ModelReference  ModelNameDialog=NEDnav.slx  SimulationMode=Normal  ModelReferenceVersion=1.2054  CopyOfModelName=NEDnav.slx  DefaultDataLogging=on
  Output Heirarchy : Subsystem
  Outputs : Outport
  Finished : Outport  Port=2
  wires:
  Model/1 -> Output Heirarchy/2(RPM)
  Model/2 -> Output Heirarchy/3(Desired Heading)
  Model/3 -> Finished/1
  Output Heirarchy/1(Outputs) -> Outputs/1
  Sensors/1 -> Bus Selector2/1, Output Heirarchy/1(Sensors)
  Bus Selector2/1 -> Model/1  "<X>"
  Bus Selector2/2 -> Model/2  "<Y>"
  Bus Selector2/3 -> Model/3  "<Heading>"
  Data Store Read3/1 -> Demux/1
  Demux/1 -> Model/4
  Demux/2 -> Model/5

== system RoboBoat_SScallv3/Main FSM/Start Speed/Gate Find and Through1/Find ==
  Sensors : Inport
  Enable : EnablePort
  Bus Selector : BusSelector  OutputSignals=Lidar Data Input.Landmarks.Distances,Lidar Data Input.Landmarks.Angles,GPS.X,GPS.Y,Compass.Heading
  MATLAB Function1 : MATLAB Function  TreatAsAtomicUnit=on
  Output Heirarchy : Subsystem
  RPM : Constant  Value=0  SampleTime=-1
  Write : DataStoreWrite  DataStoreName=GateNED
  Outputs : Outport
  Finished : Outport  Port=2
  wires:
  Output Heirarchy/1(Outputs) -> Outputs/1
  RPM/1 -> Output Heirarchy/2(RPM)
  MATLAB Function1/2(Goal) -> Write/1
  MATLAB Function1/1(found) -> Finished/1
  MATLAB Function1/3(DesiredHeading) -> Output Heirarchy/3(Desired Heading)
  Sensors/1 -> Output Heirarchy/1(Sensors), Bus Selector/1  "Sensors"
  Bus Selector/1 -> MATLAB Function1/1(Dist)  "<Distances>"
  Bus Selector/3 -> MATLAB Function1/3(X)  "<X>"
  Bus Selector/2 -> MATLAB Function1/2(Angles)  "<Angles>"
  Bus Selector/4 -> MATLAB Function1/4(Y)  "<Y>"
  Bus Selector/5 -> MATLAB Function1/5(Heading)  "<Heading>"

== system RoboBoat_SScallv3/Main FSM/Start Speed/Gate Find and Through1/Through ==
  Sensors : Inport
  Enable : EnablePort
  Bus Selector2 : BusSelector  OutputSignals=GPS.X,GPS.Y,Compass.Heading
  Data Store Read3 : DataStoreRead  DataStoreName=GateNED
  Demux : Demux  Outputs=2
  Model : ModelReference  ModelNameDialog=NEDnav.slx  SimulationMode=Normal  ModelReferenceVersion=1.2054  CopyOfModelName=NEDnav.slx  DefaultDataLogging=on
  Output Heirarchy : Subsystem
  Outputs : Outport
  Finished : Outport  Port=2
  wires:
  Model/1 -> Output Heirarchy/2(RPM)
  Model/2 -> Output Heirarchy/3(Desired Heading)
  Model/3 -> Finished/1
  Output Heirarchy/1(Outputs) -> Outputs/1
  Sensors/1 -> Bus Selector2/1, Output Heirarchy/1(Sensors)
  Bus Selector2/1 -> Model/1  "<X>"
  Bus Selector2/2 -> Model/2  "<Y>"
  Bus Selector2/3 -> Model/3  "<Heading>"
  Data Store Read3/1 -> Demux/1
  Demux/1 -> Model/4
  Demux/2 -> Model/5

== system RoboBoat_SScallv3/Sensors/Baseboard Serial/Compass Decode/Correct Heading Angle Magnetic to True North ==
  Heading Mag : Inport
  Magnetic to True North Conversion : MATLAB Function  TreatAsAtomicUnit=on
  Heading True : Outport
  wires:
  Magnetic to True North Conversion/1(HeadingT) -> Heading True/1  "Heading"
  Heading Mag/1 -> Magnetic to True North Conversion/1(HeadingM)

== system RoboBoat_SScallv3/Sinks/actuators/analog output/Subsystem ==
  Compass Heading : Inport
  Control Signals : Inport  Port=2
  Bus Creator : BusCreator  Inputs=5
  Bus Selector : BusSelector  OutputSignals=RPM,Desired Heading
  Heading Controller : Subsystem
  Propulsion Controller : Subsystem
  data log : Subsystem
  data log1 : Subsystem
  Propulsion : Outport
  Steering : Outport  Port=2
  wires:
  Bus Selector/1 -> Bus Creator/1, Propulsion Controller/1(RPM)  "<RPM>"
  Propulsion Controller/1(Propulsion) -> Propulsion/1, Bus Creator/4
  Bus Selector/2 -> Bus Creator/2, Heading Controller/1(Heading Desired)  "<Desired Heading>"
  Compass Heading/1 -> Bus Creator/3, Heading Controller/2(Compass Heading)
  Heading Controller/1(Steering) -> Steering/1, Bus Creator/5
  Bus Creator/1 -> data log/1(Sensors signal)
  Control Signals/1 -> data log1/1(Sensors signal), Bus Selector/1

== system RoboBoat_SScallv3/Main FSM/Obstacle Navigation1/Enter Gate/Gate 1 (Red & White)/Output Heirarchy ==
  Annotated Image : Inport
  Sensors : Inport  Port=2
  RPM : Inport  Port=3
  Desired Heading : Inport  Port=4
  Task Finished : Inport  Port=5
  Bus Creator : BusCreator  Inputs=3
  Bus Creator1 : BusCreator  Inputs=2
  Bus Creator2 : BusCreator  Inputs=3
  Bus Creator3 : BusCreator  Inputs=2
  Bus Creator4 : BusCreator  Inputs=2
  Due Sample Start : Constant  Value=0
  Ready to Read : Constant  Value=0
  Uno Power : Constant  Value=0
  Outputs : Outport
  wires:
  RPM/1 -> Bus Creator/1  "RPM"
  Bus Creator/1 -> Bus Creator1/1  "Control Signals"
  Bus Creator2/1 -> Bus Creator/3  "Arduino Signals"
  Uno Power/1 -> Bus Creator2/2  "Uno Power"
  Desired Heading/1 -> Bus Creator/2  "Desired Heading"
  Bus Creator1/1 -> Bus Creator4/1  "Outputs"
  Annotated Image/1 -> Bus Creator1/2  "Annotated Image"
  Sensors/1 -> Bus Creator4/2  "Sensors"
  Bus Creator4/1 -> Bus Creator3/1  "Output Signals"
  Ready to Read/1 -> Bus Creator2/1  "Ready to Read"
  Due Sample Start/1 -> Bus Creator2/3  "Due Sample Start"
  Task Finished/1 -> Bus Creator3/2  "Task Finished"
  Bus Creator3/1 -> Outputs/1

== system RoboBoat_SScallv3/Main FSM/Obstacle Navigation1/Enter Gate/Gate 2 (White & White)/Output Heirarchy ==
  Annotated Image : Inport
  Sensors : Inport  Port=2
  RPM : Inport  Port=3
  Desired Heading : Inport  Port=4
  Task Finished : Inport  Port=5
  Bus Creator : BusCreator  Inputs=3
  Bus Creator1 : BusCreator  Inputs=2
  Bus Creator2 : BusCreator  Inputs=3
  Bus Creator3 : BusCreator  Inputs=2
  Bus Creator4 : BusCreator  Inputs=2
  Due Sample Start : Constant  Value=0
  Ready to Read : Constant  Value=0
  Uno Power : Constant  Value=0
  Outputs : Outport
  wires:
  RPM/1 -> Bus Creator/1  "RPM"
  Bus Creator/1 -> Bus Creator1/1  "Control Signals"
  Bus Creator2/1 -> Bus Creator/3  "Arduino Signals"
  Uno Power/1 -> Bus Creator2/2  "Uno Power"
  Desired Heading/1 -> Bus Creator/2  "Desired Heading"
  Bus Creator1/1 -> Bus Creator4/1  "Outputs"
  Annotated Image/1 -> Bus Creator1/2  "Annotated Image"
  Sensors/1 -> Bus Creator4/2  "Sensors"
  Bus Creator4/1 -> Bus Creator3/1  "Output Signals"
  Ready to Read/1 -> Bus Creator2/1  "Ready to Read"
  Due Sample Start/1 -> Bus Creator2/3  "Due Sample Start"
  Task Finished/1 -> Bus Creator3/2  "Task Finished"
  Bus Creator3/1 -> Outputs/1

== system RoboBoat_SScallv3/Main FSM/Obstacle Navigation1/Enter Gate/Gate 3 (White & Green)/Output Heirarchy ==
  Annotated Image : Inport
  Sensors : Inport  Port=2
  RPM : Inport  Port=3
  Desired Heading : Inport  Port=4
  Task Finished : Inport  Port=5
  Bus Creator : BusCreator  Inputs=3
  Bus Creator1 : BusCreator  Inputs=2
  Bus Creator2 : BusCreator  Inputs=3
  Bus Creator3 : BusCreator  Inputs=2
  Bus Creator4 : BusCreator  Inputs=2
  Due Sample Start : Constant  Value=0
  Ready to Read : Constant  Value=0
  Uno Power : Constant  Value=0
  Outputs : Outport
  wires:
  RPM/1 -> Bus Creator/1  "RPM"
  Bus Creator/1 -> Bus Creator1/1  "Control Signals"
  Bus Creator2/1 -> Bus Creator/3  "Arduino Signals"
  Uno Power/1 -> Bus Creator2/2  "Uno Power"
  Desired Heading/1 -> Bus Creator/2  "Desired Heading"
  Bus Creator1/1 -> Bus Creator4/1  "Outputs"
  Annotated Image/1 -> Bus Creator1/2  "Annotated Image"
  Sensors/1 -> Bus Creator4/2  "Sensors"
  Bus Creator4/1 -> Bus Creator3/1  "Output Signals"
  Ready to Read/1 -> Bus Creator2/1  "Ready to Read"
  Due Sample Start/1 -> Bus Creator2/3  "Due Sample Start"
  Task Finished/1 -> Bus Creator3/2  "Task Finished"
  Bus Creator3/1 -> Outputs/1

== system RoboBoat_SScallv3/Main FSM/Obstacle Navigation1/Exit Gate/Gate 1 (Red & White)/Output Heirarchy ==
  Annotated Image : Inport
  Sensors : Inport  Port=2
  RPM : Inport  Port=3
  Desired Heading : Inport  Port=4
  Task Finished : Inport  Port=5
  Bus Creator : BusCreator  Inputs=3
  Bus Creator1 : BusCreator  Inputs=2
  Bus Creator2 : BusCreator  Inputs=3
  Bus Creator3 : BusCreator  Inputs=2
  Bus Creator4 : BusCreator  Inputs=2
  Due Sample Start : Constant  Value=0
  Ready to Read : Constant  Value=0
  Uno Power : Constant  Value=0
  Outputs : Outport
  wires:
  RPM/1 -> Bus Creator/1  "RPM"
  Bus Creator/1 -> Bus Creator1/1  "Control Signals"
  Bus Creator2/1 -> Bus Creator/3  "Arduino Signals"
  Uno Power/1 -> Bus Creator2/2  "Uno Power"
  Desired Heading/1 -> Bus Creator/2  "Desired Heading"
  Bus Creator1/1 -> Bus Creator4/1  "Outputs"
  Annotated Image/1 -> Bus Creator1/2  "Annotated Image"
  Sensors/1 -> Bus Creator4/2  "Sensors"
  Bus Creator4/1 -> Bus Creator3/1  "Output Signals"
  Ready to Read/1 -> Bus Creator2/1  "Ready to Read"
  Due Sample Start/1 -> Bus Creator2/3  "Due Sample Start"
  Task Finished/1 -> Bus Creator3/2  "Task Finished"
  Bus Creator3/1 -> Outputs/1

== system RoboBoat_SScallv3/Main FSM/Obstacle Navigation1/Exit Gate/Gate 2 (White & White)/Output Heirarchy ==
  Annotated Image : Inport
  Sensors : Inport  Port=2
  RPM : Inport  Port=3
  Desired Heading : Inport  Port=4
  Task Finished : Inport  Port=5
  Bus Creator : BusCreator  Inputs=3
  Bus Creator1 : BusCreator  Inputs=2
  Bus Creator2 : BusCreator  Inputs=3
  Bus Creator3 : BusCreator  Inputs=2
  Bus Creator4 : BusCreator  Inputs=2
  Due Sample Start : Constant  Value=0
  Ready to Read : Constant  Value=0
  Uno Power : Constant  Value=0
  Outputs : Outport
  wires:
  RPM/1 -> Bus Creator/1  "RPM"
  Bus Creator/1 -> Bus Creator1/1  "Control Signals"
  Bus Creator2/1 -> Bus Creator/3  "Arduino Signals"
  Uno Power/1 -> Bus Creator2/2  "Uno Power"
  Desired Heading/1 -> Bus Creator/2  "Desired Heading"
  Bus Creator1/1 -> Bus Creator4/1  "Outputs"
  Annotated Image/1 -> Bus Creator1/2  "Annotated Image"
  Sensors/1 -> Bus Creator4/2  "Sensors"
  Bus Creator4/1 -> Bus Creator3/1  "Output Signals"
  Ready to Read/1 -> Bus Creator2/1  "Ready to Read"
  Due Sample Start/1 -> Bus Creator2/3  "Due Sample Start"
  Task Finished/1 -> Bus Creator3/2  "Task Finished"
  Bus Creator3/1 -> Outputs/1

== system RoboBoat_SScallv3/Main FSM/Obstacle Navigation1/Exit Gate/Gate 3 (White & Green)/Output Heirarchy ==
  Annotated Image : Inport
  Sensors : Inport  Port=2
  RPM : Inport  Port=3
  Desired Heading : Inport  Port=4
  Task Finished : Inport  Port=5
  Bus Creator : BusCreator  Inputs=3
  Bus Creator1 : BusCreator  Inputs=2
  Bus Creator2 : BusCreator  Inputs=3
  Bus Creator3 : BusCreator  Inputs=2
  Bus Creator4 : BusCreator  Inputs=2
  Due Sample Start : Constant  Value=0
  Ready to Read : Constant  Value=0
  Uno Power : Constant  Value=0
  Outputs : Outport
  wires:
  RPM/1 -> Bus Creator/1  "RPM"
  Bus Creator/1 -> Bus Creator1/1  "Control Signals"
  Bus Creator2/1 -> Bus Creator/3  "Arduino Signals"
  Uno Power/1 -> Bus Creator2/2  "Uno Power"
  Desired Heading/1 -> Bus Creator/2  "Desired Heading"
  Bus Creator1/1 -> Bus Creator4/1  "Outputs"
  Annotated Image/1 -> Bus Creator1/2  "Annotated Image"
  Sensors/1 -> Bus Creator4/2  "Sensors"
  Bus Creator4/1 -> Bus Creator3/1  "Output Signals"
  Ready to Read/1 -> Bus Creator2/1  "Ready to Read"
  Due Sample Start/1 -> Bus Creator2/3  "Due Sample Start"
  Task Finished/1 -> Bus Creator3/2  "Task Finished"
  Bus Creator3/1 -> Outputs/1
